simulink library "LumpedParameterLiftModels"  (R2021b)
settings: Solver=VariableStepAuto  StartTime=0.0  StopTime=10.0  RelTol=1e-3
values from neighbouring files (symbols this model uses):
  x0 = x_eq    [test_LiftDynamicsEquation.m]    (also in test_discretization.m)
libraries: $bdroot x5, simulink x2
settings Model: Creator=manue  LastModifiedBy=manue

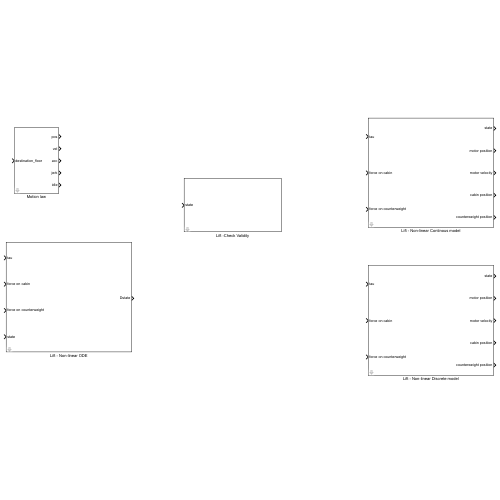
[thumbnail: Simulink's stored preview of the top-level diagram]
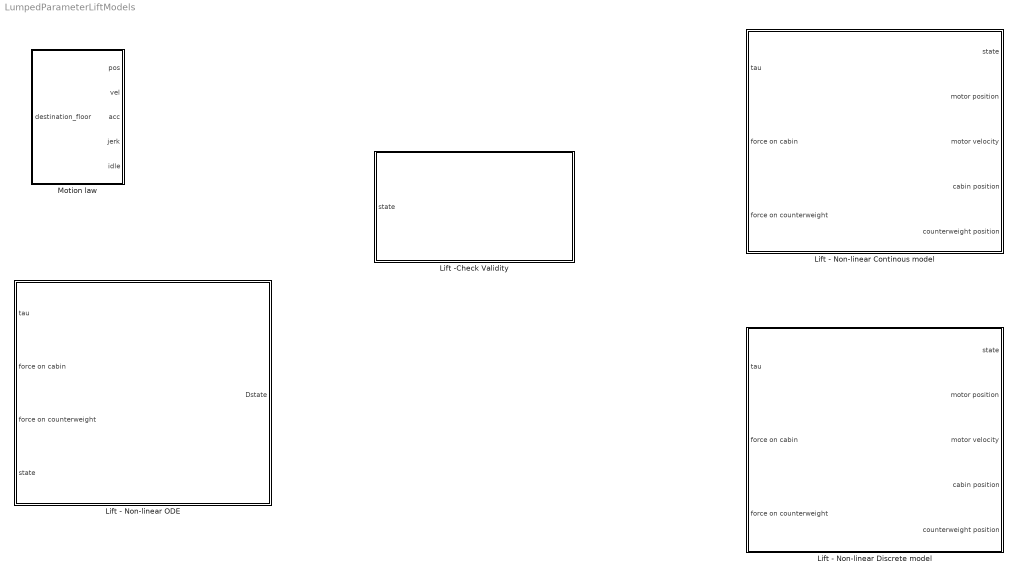
== system LumpedParameterLiftModels ==
  Lift - Non-linear Continous model : Subsystem  mask{Jp=1, Jm=0.1, Mc=600, Mw=650, LinearStiffness=2100000, LinearDamping=30, Rp=0.5, mu=0.8, BuildingHeight=30, MotorViscousFriction=0, g=9.806, gearbox=1, min_length=3, x9_init=0}
      mask prompts: Jp "Pulley inertia"; Jm "motor inertia"; Mc "Cabin mass"; Mw "Counterweight mass"; LinearStiffness "stiffness of 1 meter of rope"; LinearDamping "damping of 1 meter of rope"; Rp "Pulley radius"; mu "Linear Density"; BuildingHeight "Building Height"; MotorViscousFriction "Motor Viscous Friction"; g "gravitational acceleration"; gearbox "Gearbox ratio"; min_length "Minimum distance between pulley and cabin"; x9_init "Initial motor position"
      mask help:
      | Elastic model of the list, using continuous integrator.
      | Initial conditions are computed at the startup using the Initial motor position to initialize the other states at the equilibrium.
      mask init:
      | [x0] = LiftEquilibrium(BuildingHeight,LinearStiffness,Mc,Mw,Rp,0,0,g,gearbox,min_length,mu,x9_init);
  Lift - Non-linear Discrete model : Subsystem  mask{Jp=1, Jm=0.1, Mc=600, Mw=650, LinearStiffness=2100000, LinearDamping=30, Rp=0.5, mu=0.8, BuildingHeight=30, MotorViscousFriction=0, g=9.806, gearbox=1, min_length=3, x9_init=0, Ts=1e-3}
      mask prompts: Jp "Pulley inertia"; Jm "motor inertia"; Mc "Cabin mass"; Mw "Counterweight mass"; LinearStiffness "stiffness of 1 meter of rope"; LinearDamping "damping of 1 meter of rope"; Rp "Pulley radius"; mu "Linear Density"; BuildingHeight "Building Height"; MotorViscousFriction "Motor Viscous Friction"; g "gravitational acceleration"; gearbox "Gearbox ratio"; min_length "Minimum distance between pulley and cabin"; x9_init "Initial motor position"; Ts "Sample time"
      mask help:
      | Elastic model of the list, using continuous integrator.
      | Initial conditions are computed at the startup using the Initial motor position to initialize the other states at the equilibrium.
      mask init:
      | [x0] = LiftEquilibrium(BuildingHeight,LinearStiffness,Mc,Mw,Rp,0,0,g,gearbox,min_length,mu,x9_init);
  Lift - Non-linear ODE : Subsystem  mask{Jp=1, Jm=0.1, Mc=600, Mw=650, LinearStiffness=2100000, LinearDamping=30, Rp=0.5, mu=0.8, BuildingHeight=30, MotorViscousFriction=0, g=9.806, gearbox=1, min_length=3}
      mask prompts: Jp "Pulley inertia"; Jm "motor inertia"; Mc "Cabin mass"; Mw "Counterweight mass"; LinearStiffness "stiffness of 1 meter of rope"; LinearDamping "damping of 1 meter of rope"; Rp "Pulley radius"; mu "Linear Density"; BuildingHeight "Building Height"; MotorViscousFriction "Motor Viscous Friction"; g "gravitational acceleration"; gearbox "Gearbox ratio"; min_length "Minimum distance between pulley and cabin"
      mask help:
      | Elastic model of the list, using continuous integrator.
      | Initial conditions are computed at the startup using the Initial motor position to initialize the other states at the equilibrium.
  Lift -Check Validity : Subsystem  mask{BuildingHeight=30, min_length=3}
      mask prompts: BuildingHeight "Building Height"; min_length "Minimum distance between pulley and cabin"
      mask help:
      | Elastic model of the list, using continuous integrator.
      | Initial conditions are computed at the startup using the Initial motor position to initialize the other states at the equilibrium.
  Motion law : Subsystem  mask(Lift motion law generator){MaxVel=1, MaxAcc=10, MaxJerk=100, Ts=0.002, floor_height=3}
      mask prompts: MaxVel "Maximum Velocity"; MaxAcc "Maximum Acceleration"; MaxJerk "Maximum Jerk"; Ts "Sample period"; floor_height "Floor height"
      mask help: idle is true when no motion law is applied

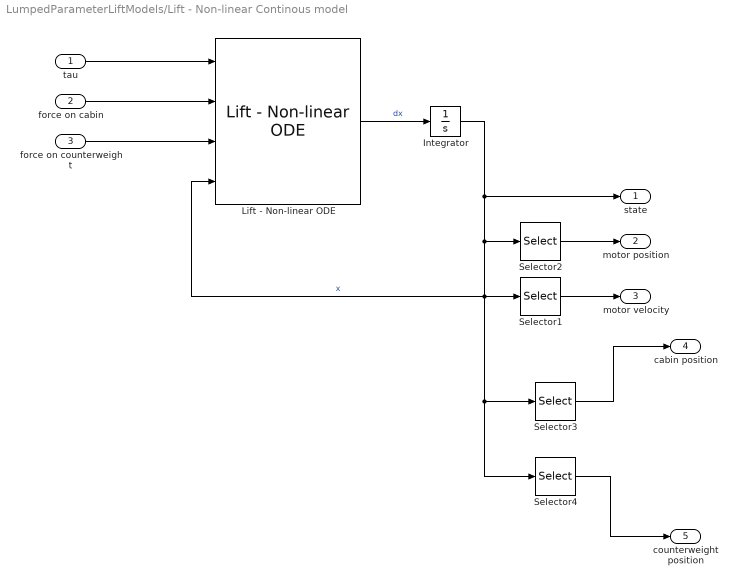
== system LumpedParameterLiftModels/Lift - Non-linear Continous model ==
  tau : Inport
  force on cabin : Inport  Port=2
  force on counterweight : Inport  Port=3
  Integrator : Integrator  InitialCondition=x0
  Lift - Non-linear ODE : $bdroot/Lift - Non-linear ODE  Jp=Jp  Jm=Jm  Mc=Mc  Mw=Mw  LinearStiffness=LinearStiffness  LinearDamping=LinearDamping  Rp=Rp  mu=mu  BuildingHeight=BuildingHeight  MotorViscousFriction=MotorViscousFriction  g=g  gearbox=gearbox  min_length=min_length
  Selector1 : Selector  InputPortWidth=10  IndexOptions=Index vector (dialog)  Indices=[10]  OutputSizes=1
  Selector2 : Selector  InputPortWidth=10  IndexOptions=Index vector (dialog)  Indices=[9]  OutputSizes=1
  Selector3 : Selector  InputPortWidth=10  IndexOptions=Index vector (dialog)  Indices=[7]  OutputSizes=1
  Selector4 : Selector  InputPortWidth=10  IndexOptions=Index vector (dialog)  Indices=[1]  OutputSizes=1
  state : Outport
  motor position : Outport  Port=2
  motor velocity : Outport  Port=3
  cabin position : Outport  Port=4
  counterweight position : Outport  Port=5
  wires:
  Lift - Non-linear ODE/1 -> Integrator/1  "dx"
  Integrator/1 -> Lift - Non-linear ODE/4, Selector3/1, Selector4/1, Selector1/1, Selector2/1, state/1  "x"
  Selector2/1 -> motor position/1
  Selector1/1 -> motor velocity/1
  Selector3/1 -> cabin position/1
  Selector4/1 -> counterweight position/1
  force on counterweight/1 -> Lift - Non-linear ODE/3
  force on cabin/1 -> Lift - Non-linear ODE/2
  tau/1 -> Lift - Non-linear ODE/1

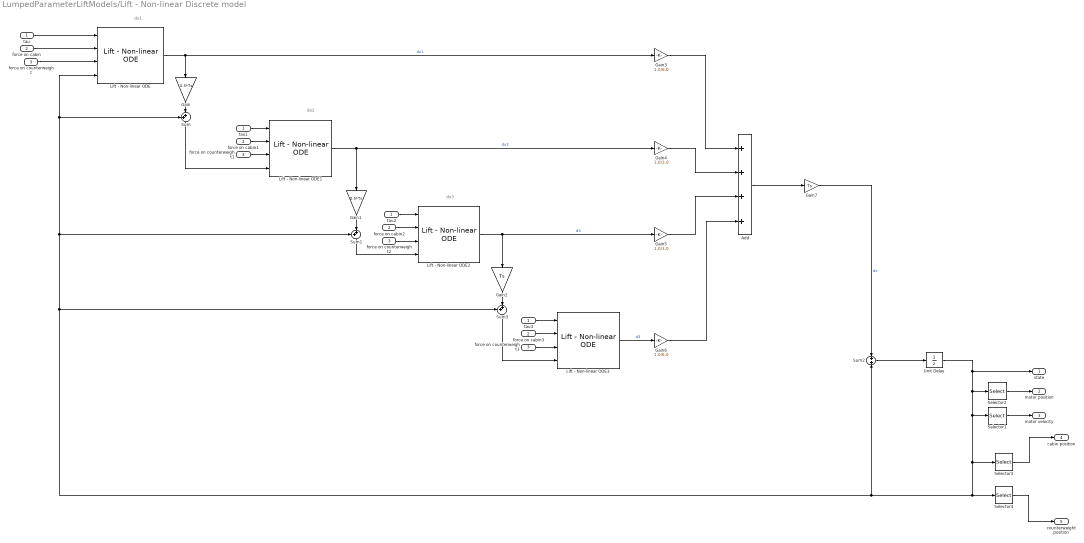
== system LumpedParameterLiftModels/Lift - Non-linear Discrete model ==
  note: dx3
  note: dx2
  note: dx1
  tau : Inport
  force on cabin : Inport  Port=2
  force on counterweight : Inport  Port=3
  Add : Sum  Inputs=++++
  Gain : Gain  Gain=0.5*Ts
  Gain1 : Gain  Gain=0.5*Ts
  Gain2 : Gain  Gain=Ts
  Gain3 : Gain  Gain=1.0/6.0
  Gain4 : Gain  Gain=1.0/3.0
  Gain5 : Gain  Gain=1.0/3.0
  Gain6 : Gain  Gain=1.0/6.0
  Gain7 : Gain  Gain=Ts
  Lift - Non-linear ODE{,1..3} (4 alike) : $bdroot/Lift - Non-linear ODE  Jp=Jp  Jm=Jm  Mc=Mc  Mw=Mw  LinearStiffness=LinearStiffness  LinearDamping=LinearDamping  Rp=Rp  mu=mu  BuildingHeight=BuildingHeight  MotorViscousFriction=MotorViscousFriction  g=g  gearbox=gearbox  min_length=min_length
  Selector1 : Selector  InputPortWidth=10  IndexOptions=Index vector (dialog)  Indices=[10]  OutputSizes=1
  Selector2 : Selector  InputPortWidth=10  IndexOptions=Index vector (dialog)  Indices=[9]  OutputSizes=1
  Selector3 : Selector  InputPortWidth=10  IndexOptions=Index vector (dialog)  Indices=[7]  OutputSizes=1
  Selector4 : Selector  InputPortWidth=10  IndexOptions=Index vector (dialog)  Indices=[1]  OutputSizes=1
  Sum : Sum  Inputs=++|
  Sum1 : Sum  Inputs=++|
  Sum2 : Sum
  Sum3 : Sum  Inputs=++|
  Unit Delay : UnitDelay  InitialCondition=x0  SampleTime=Ts  HasFrameUpgradeWarning=on
  force on cabin1 : InportShadow  Port=2
  force on cabin2 : InportShadow  Port=2
  force on cabin3 : InportShadow  Port=2
  force on counterweight1 : InportShadow  Port=3
  force on counterweight2 : InportShadow  Port=3
  force on counterweight3 : InportShadow  Port=3
  tau1 : InportShadow
  tau2 : InportShadow
  tau3 : InportShadow
  state : Outport
  motor position : Outport  Port=2
  motor velocity : Outport  Port=3
  cabin position : Outport  Port=4
  counterweight position : Outport  Port=5
  wires:
  tau/1 -> Lift - Non-linear ODE/1
  force on cabin/1 -> Lift - Non-linear ODE/2
  force on counterweight/1 -> Lift - Non-linear ODE/3
  Selector4/1 -> counterweight position/1
  Selector3/1 -> cabin position/1
  Selector1/1 -> motor velocity/1
  Selector2/1 -> motor position/1
  Lift - Non-linear ODE/1 -> Gain3/1, Gain/1  "dx1"
  Gain/1 -> Sum/2
  Sum/1 -> Lift - Non-linear ODE1/4
  tau1/1 -> Lift - Non-linear ODE1/1
  force on cabin1/1 -> Lift - Non-linear ODE1/2
  force on counterweight1/1 -> Lift - Non-linear ODE1/3
  Lift - Non-linear ODE1/1 -> Gain4/1, Gain1/1  "dx2"
  Gain1/1 -> Sum1/2
  Sum1/1 -> Lift - Non-linear ODE2/4
  tau2/1 -> Lift - Non-linear ODE2/1
  force on cabin2/1 -> Lift - Non-linear ODE2/2
  force on counterweight2/1 -> Lift - Non-linear ODE2/3
  Lift - Non-linear ODE2/1 -> Gain5/1, Gain2/1  "d3"
  Unit Delay/1 -> state/1, Selector2/1, Selector1/1, Selector4/1, Sum2/2, Sum3/1, Sum1/1, Sum/1, Lift - Non-linear ODE/4, Selector3/1
  Gain2/1 -> Sum3/2
  Sum3/1 -> Lift - Non-linear ODE3/4
  tau3/1 -> Lift - Non-linear ODE3/1
  force on cabin3/1 -> Lift - Non-linear ODE3/2
  force on counterweight3/1 -> Lift - Non-linear ODE3/3
  Lift - Non-linear ODE3/1 -> Gain6/1  "d3"
  Gain4/1 -> Add/2
  Gain5/1 -> Add/3
  Gain3/1 -> Add/1
  Gain6/1 -> Add/4
  Add/1 -> Gain7/1
  Gain7/1 -> Sum2/1  "dx"
  Sum2/1 -> Unit Delay/1

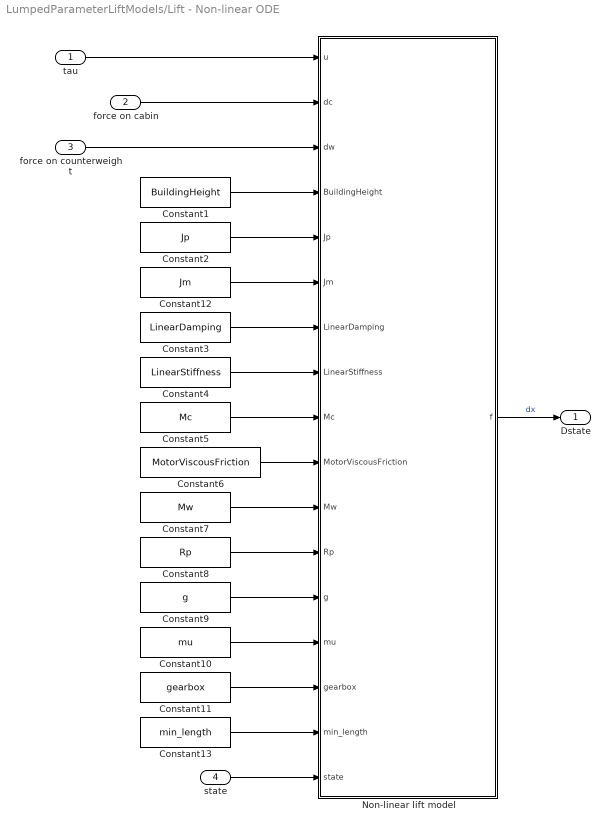
== system LumpedParameterLiftModels/Lift - Non-linear ODE ==
  tau : Inport
  force on cabin : Inport  Port=2
  force on counterweight : Inport  Port=3
  state : Inport  Port=4
  Constant1 : Constant  Value=BuildingHeight
  Constant10 : Constant  Value=mu
  Constant11 : Constant  Value=gearbox
  Constant12 : Constant  Value=Jm
  Constant13 : Constant  Value=min_length
  Constant2 : Constant  Value=Jp
  Constant3 : Constant  Value=LinearDamping
  Constant4 : Constant  Value=LinearStiffness
  Constant5 : Constant  Value=Mc
  Constant6 : Constant  Value=MotorViscousFriction
  Constant7 : Constant  Value=Mw
  Constant8 : Constant  Value=Rp
  Constant9 : Constant  Value=g
  Non-linear lift model : MATLAB Function  TreatAsAtomicUnit=on
  Dstate : Outport
  wires:
  Constant13/1 -> Non-linear lift model/16(min_length)
  Constant11/1 -> Non-linear lift model/15(gearbox)
  Constant6/1 -> Non-linear lift model/10(MotorViscousFriction)
  Constant12/1 -> Non-linear lift model/6(Jm)
  Constant2/1 -> Non-linear lift model/5(Jp)
  Constant10/1 -> Non-linear lift model/14(mu)
  Constant9/1 -> Non-linear lift model/13(g)
  Constant8/1 -> Non-linear lift model/12(Rp)
  Constant7/1 -> Non-linear lift model/11(Mw)
  Constant5/1 -> Non-linear lift model/9(Mc)
  Constant4/1 -> Non-linear lift model/8(LinearStiffness)
  Constant3/1 -> Non-linear lift model/7(LinearDamping)
  Constant1/1 -> Non-linear lift model/4(BuildingHeight)
  force on counterweight/1 -> Non-linear lift model/3(dw)
  force on cabin/1 -> Non-linear lift model/2(dc)
  tau/1 -> Non-linear lift model/1(u)
  Non-linear lift model/1(f) -> Dstate/1  "dx"
  state/1 -> Non-linear lift model/17(state)

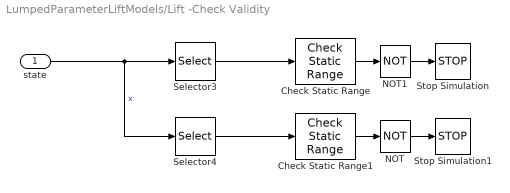
== system LumpedParameterLiftModels/Lift -Check Validity ==
  state : Inport
  Check Static Range : simulink/Model Verification/Check  Static Range  Description=-min_length*.9 <= u <= BuildingHeight+min_length*.9  max=BuildingHeight+min_length*.9  max_included=on  min=-min_length*.9  min_included=on  enabled=on  stopWhenAssertionFail=on  export=on  icon=graphic
      settings: SourceProductBaseCode=SL
  Check Static Range1 : simulink/Model Verification/Check  Static Range  Description=-min_length*.9 <= u <= BuildingHeight+min_length*.9  max=BuildingHeight+min_length*.9  max_included=on  min=-min_length*.9  min_included=on  enabled=on  stopWhenAssertionFail=on  export=on  icon=graphic
      settings: SourceProductBaseCode=SL
  NOT : Logic  Operator=NOT  IconShape=distinctive  AllPortsSameDT=off  OutDataTypeStr=boolean
  NOT1 : Logic  Operator=NOT  IconShape=distinctive  AllPortsSameDT=off  OutDataTypeStr=boolean
  Selector3 : Selector  InputPortWidth=10  IndexOptions=Index vector (dialog)  Indices=[7]  OutputSizes=1
  Selector4 : Selector  InputPortWidth=10  IndexOptions=Index vector (dialog)  Indices=[1]  OutputSizes=1
  Stop Simulation : Stop
  Stop Simulation1 : Stop
  wires:
  NOT1/1 -> Stop Simulation/1
  NOT/1 -> Stop Simulation1/1
  Check Static Range1/1 -> NOT/1
  Check Static Range/1 -> NOT1/1
  Selector4/1 -> Check Static Range1/1
  Selector3/1 -> Check Static Range/1
  state/1 -> Selector4/1, Selector3/1  "x"

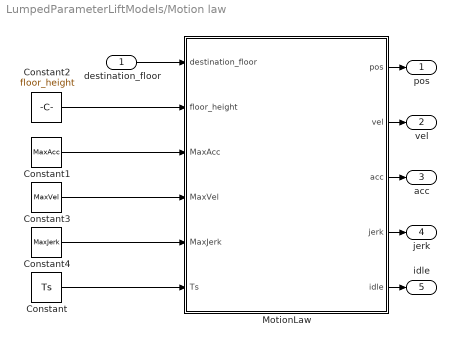
== system LumpedParameterLiftModels/Motion law ==
  destination_floor : Inport
  Constant : Constant  Value=Ts
  Constant1 : Constant  Value=MaxAcc
  Constant2 : Constant  Value=floor_height
  Constant3 : Constant  Value=MaxVel
  Constant4 : Constant  Value=MaxJerk
  MotionLaw : MATLAB Function  TreatAsAtomicUnit=on  SystemSampleTime=Ts
  pos : Outport
  vel : Outport  Port=2
  acc : Outport  Port=3
  jerk : Outport  Port=4
  idle : Outport  Port=5
  wires:
  Constant3/1 -> MotionLaw/4(MaxVel)
  MotionLaw/4(jerk) -> jerk/1
  destination_floor/1 -> MotionLaw/1(destination_floor)
  Constant4/1 -> MotionLaw/5(MaxJerk)
  Constant2/1 -> MotionLaw/2(floor_height)
  Constant1/1 -> MotionLaw/3(MaxAcc)
  Constant/1 -> MotionLaw/6(Ts)
  MotionLaw/2(vel) -> vel/1
  MotionLaw/5(idle) -> idle/1
  MotionLaw/1(pos) -> pos/1
  MotionLaw/3(acc) -> acc/1

== matlab function LumpedParameterLiftModels/Lift - Non-linear ODE/Non-linear lift model ==
  data: u input; dc input; dw input; BuildingHeight input; Jp input; Jm input; LinearDamping input; LinearStiffness input; Mc input; MotorViscousFriction input; Mw input; Rp input; g input; mu input; gearbox input; min_length input; state input; f output
function f = LiftDynamicsEquation(u,dc,dw,BuildingHeight,Jp,Jm,LinearDamping,LinearStiffness,Mc,MotorViscousFriction,Mw,Rp,g,mu,gearbox,min_length,state)
%    This function was generated by the Symbolic Math Toolbox version 9.0.
%    27-Oct-2022 19:13:42

%Version: 1.0
t2 = Rp.^2;
t3 = gearbox.^2;
t4 = min_length.^2;
t5 = state(9).^2;
t6 = LinearStiffness.*min_length.*2.0;
t7 = Rp.*gearbox.*state(9);
t8 = 1.0./mu;
t9 = BuildingHeight.*LinearStiffness.*2.0;
t10 = min_length./2.0;
t11 = g.*mu.*t4;
t12 = min_length+t7;
t13 = t7./2.0;
t16 = g.*mu.*t2.*t3.*t5;
t14 = -t11;
t15 = 1.0./t12;
t17 = t10+t13;
t18 = 1.0./t17;
mt1 = [state(2);-(dw+Mw.*g+LinearStiffness.*t18.*(state(1)-state(3)+t17)+LinearDamping.*t18.*(state(2)-state(4)+gearbox.*state(10).*(3.0./2.0)))./Mw;state(4);t8.*t15.^2.*(t6+t9+t14-t16+LinearDamping.*state(2).*2.0-LinearDamping.*state(4).*4.0+LinearStiffness.*state(1).*2.0-LinearStiffness.*state(3).*4.0+LinearDamping.*gearbox.*state(10).*4.0-g.*min_length.*mu.*t7.*2.0);state(6);(t8.*t15.*(t6+t9+t14+t16-LinearDamping.*state(6).*4.0+LinearDamping.*state(8).*2.0-LinearStiffness.*state(5).*4.0+LinearStiffness.*state(7).*2.0-BuildingHeight.*g.*min_length.*mu-BuildingHeight.*g.*mu.*t7))./(BuildingHeight+min_length-t7);state(8);-(dc+Mc.*g+LinearStiffness.*t18.*(BuildingHeight./2.0-state(5)+state(7)+t10-t13)-LinearDamping.*t18.*(state(6)-state(8)+(gearbox.*state(10))./2.0))./Mc;state(10)];
mt2 = [(t15.*(min_length.*u+t7.*u-MotorViscousFriction.*min_length.*state(10)-MotorViscousFriction.*state(10).*t7-LinearStiffness.*state(9).*t2.*t3.*2.0+BuildingHeight.*LinearStiffness.*Rp.*gearbox-LinearDamping.*Rp.*gearbox.*state(4).*2.0+LinearDamping.*Rp.*gearbox.*state(6).*2.0-LinearStiffness.*Rp.*gearbox.*state(3).*2.0+LinearStiffness.*Rp.*gearbox.*state(5).*2.0))./(Jm+Jp.*t3)];
f = [mt1;mt2];

== matlab function LumpedParameterLiftModels/Motion law/MotionLaw ==
  data: destination_floor input; floor_height input; MaxAcc input; MaxVel input; MaxJerk input; Ts input; pos output; vel output; acc output; jerk output; idle output
function [pos,vel,acc,jerk,idle]  = MotionLawStateMachine(destination_floor,floor_height,MaxAcc,MaxVel,MaxJerk,Ts)

persistent state last_floor time duration direction t1 t2 t4 destination_floor_
if isempty(state)
    state=0; %IDLE
    last_floor=destination_floor;
    destination_floor_=destination_floor;
    time=0;
    duration=1;
    direction=0;
    t1=0;
    t2=0;
    t4=0;

end


idle=false;


if (state==0) && (destination_floor~=last_floor)
    state=1; % TRANSITION
    time=0;
    CruiseVel=MaxVel;
    destination_floor_=destination_floor;
    distance=abs(destination_floor-last_floor)*floor_height;


    direction=sign(destination_floor-last_floor);


    if MaxVel>MaxAcc^2/(2*MaxJerk)
        %case 1
        limit_distance_case1=(MaxVel*(MaxAcc^2 + MaxVel*MaxJerk))/(MaxAcc*MaxJerk);


        if (distance>limit_distance_case1)
            % case 1.1
            CruiseVel=MaxVel;
            law_case=11;
        else
            CruiseVel=-(MaxAcc^2 - MaxAcc^(1/2)*(MaxAcc^3 + 4*distance*MaxJerk^2)^(1/2))/(2*MaxJerk);

            if CruiseVel>MaxAcc^2/(2*MaxJerk)
                %case 1.2
                law_case=12;
            else
                limit_distance_case2=(2*CruiseVel^(3/2))/MaxJerk^(1/2);
                if distance>limit_distance_case2
                    law_case=21;
                else
                    law_case=22;
                end
            end
        end

    else
        limit_distance_case2=(2*MaxVel^(3/2))/MaxJerk^(1/2);
        if distance>limit_distance_case2
            law_case=21;
        else
            law_case=22;
        end
    end

    switch law_case
        case 11
            t1=MaxAcc/MaxJerk;
            t2=(- MaxAcc^2/MaxJerk + MaxVel)/MaxAcc;
            t4=(distance - (MaxVel*(MaxAcc^2 + MaxVel*MaxJerk))/(MaxAcc*MaxJerk))/MaxVel;
            CruiseVel=MaxVel;
        case 12
            t1=MaxAcc/MaxJerk;
            CruiseVel=-(MaxAcc^2 - MaxAcc^(1/2)*(MaxAcc^3 + 4*distance*MaxJerk^2)^(1/2))/(2*MaxJerk);
            t2=-(3*MaxAcc^(3/2) - (MaxAcc^3 + 4*distance*MaxJerk^2)^(1/2))/(2*MaxAcc^(1/2)*MaxJerk);
            t4=0;
        case 21
            %CruiseVel=MaxVel;
            t1=CruiseVel^(1/2)/MaxJerk^(1/2);
            t2=0;
            t4=(distance - (2*CruiseVel^(3/2))/MaxJerk^(1/2))/CruiseVel;

        otherwise % case 22
            CruiseVel=((MaxJerk^(1/2)*distance)/2)^(2/3);
            t1=CruiseVel^(1/2)/MaxJerk^(1/2);
            t2=0;
            t4=0;
    end
    duration=4*t1+2*t2+t4; % t1+t2+t3+t4+t5+t6+t7, t1=t3=t5=t6,t2=t6
elseif (state==1) && (time>=duration)
    state=0;
    last_floor=destination_floor_;
end

if (state==0)
    
    idle=true;
    pos=last_floor*floor_height;
    vel=0;
    acc=0;
    jerk=0;
else%if (state==1)
    time=time+Ts;
    [jerk,acc,vel,pos]=JerkMotionLaw(MaxJerk,t1,t2,t4,time)   ;
    if direction>0
        pos=last_floor*floor_height+pos;
    else
        pos=last_floor*floor_height-pos;
        vel=-vel;
        acc=-acc;
        jerk=-jerk;
    end
    idle=false;
end

end

function [jerk,acc,vel,pos]=JerkMotionLaw(MaxJerk,t1,t2,t4,time)   

if (time<t1)
	jerk=MaxJerk;
	acc=MaxJerk*time;
	vel=(MaxJerk*time^2)/2;
	pos=(MaxJerk*time^3)/6;
elseif (time<t1 + t2)
	jerk=0;
	acc=MaxJerk*t1;
	vel=(MaxJerk*t1^2)/2 - MaxJerk*t1*(t1 - time);
	pos=(MaxJerk*t1^3)/6 - (MaxJerk*t1*time*(t1 - time))/2;
elseif (time<2*t1 + t2)
	jerk=-MaxJerk;
	acc=MaxJerk*t1 + MaxJerk*(t1 + t2 - time);
	vel=(MaxJerk*t1*(t1 + 2*t2))/2 - (MaxJerk*(4*t1*t2 - 4*t1*time - 2*t2*time + 3*t1^2 + t2^2 + time^2))/2;
	pos=(MaxJerk*t1^3)/6 - (MaxJerk*(t1 + t2 - time)*(t1*t2 + 5*t1*time + 2*t2*time - t1^2 - t2^2 - time^2))/6 + (MaxJerk*t1*t2*(t1 + t2))/2;
elseif (time<2*t1 + t2 + t4)
	jerk=0;
	acc=0;
	vel=MaxJerk*t1*(t1 + t2);
	pos=(MaxJerk*t1*(3*t1*t2 + 2*t1^2 + t2^2))/2 - MaxJerk*t1*(t1 + t2)*(2*t1 + t2 - time);
elseif (time<3*t1 + t2 + t4)
	jerk=-MaxJerk;
	acc=MaxJerk*(2*t1 + t2 + t4 - time);
	vel=MaxJerk*t1*(t1 + t2) - (MaxJerk*(2*t1 + t2 + t4 - time)^2)/2;
	pos=(MaxJerk*t1*(t1 + t2)*(2*t1 + t2 + 2*t4))/2 - (MaxJerk*(2*t1 + t2 + t4 - time)*(2*t1*t2 - 4*t1*t4 - 2*t2*t4 + 4*t1*time + 2*t2*time + 2*t4*time + 2*t1^2 - t2^2 - t4^2 - time^2))/6;
elseif (time<3*t1 + 2*t2 + t4)
	jerk=0;
	acc=-MaxJerk*t1;
	vel=MaxJerk*t1*(3*t1 + t2 + t4 - time) + (MaxJerk*t1*(t1 + 2*t2))/2;
	pos=(MaxJerk*t1*(15*t1*t2 + 6*t1*t4 + 6*t2*t4 + 11*t1^2 + 3*t2^2))/6 - (MaxJerk*t1*(13*t1*t2 + 7*t1*t4 + 4*t2*t4 - 7*t1*time - 4*t2*time - 2*t4*time + 12*t1^2 + 3*t2^2 + t4^2 + time^2))/2;
elseif (time<4*t1 + 2*t2 + t4)
	jerk=MaxJerk;
	acc=- MaxJerk*t1 - MaxJerk*(3*t1 + 2*t2 + t4 - time);
	vel=(MaxJerk*t1^2)/2 + (MaxJerk*(16*t1*t2 + 8*t1*t4 + 4*t2*t4 - 8*t1*time - 4*t2*time - 2*t4*time + 15*t1^2 + 4*t2^2 + t4^2 + time^2))/2;
	pos=(MaxJerk*t1*(18*t1*t2 + 6*t1*t4 + 6*t2*t4 + 11*t1^2 + 6*t2^2))/6 - (MaxJerk*(48*t1*t2^2 + 96*t1^2*t2 + 12*t1*t4^2 + 48*t1^2*t4 + 6*t2*t4^2 + 12*t2^2*t4 + 12*t1*time^2 - 48*t1^2*time + 6*t2*time^2 - 12*t2^2*time + 3*t4*time^2 - 3*t4^2*time + 63*t1^3 + 8*t2^3 + t4^3 - time^3 + 48*t1*t2*t4 - 48*t1*t2*time - 24*t1*t4*time - 12*t2*t4*time))/6;
else
	jerk=0;
	acc=0;
	vel=0;
	pos=MaxJerk*t1*(t1 + t2)*(2*t1 + t2 + t4);
end
end
